simulink model "system2_frequency"  (R2019b)
settings: Solver=VariableStepAuto  StartTime=0.0  StopTime=10.0  RelTol=1e-3
settings Model: Creator=davis  LastModifiedBy=davis

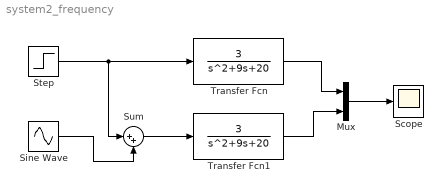
== system system2_frequency ==
  Mux : Mux  Inputs=2
  Scope : Scope
  Sine Wave : Sin  SampleTime=0
  Step : Step  Time=0  SampleTime=0
  Sum : Sum  Inputs=|++
  Transfer Fcn : TransferFcn  Numerator=[3]  Denominator=[1 9 20]
  Transfer Fcn1 : TransferFcn  Numerator=[3]  Denominator=[1 9 20]
  wires:
  Sine Wave/1 -> Sum/2
  Step/1 -> Sum/1, Transfer Fcn/1
  Transfer Fcn/1 -> Mux/1
  Mux/1 -> Scope/1
  Sum/1 -> Transfer Fcn1/1
  Transfer Fcn1/1 -> Mux/2
